simulink model "bh_smd_MAIN_simple"  (R2018a)
settings: configuration reference "CF_01" (kept outside this file)
settings Model: DataDictionary=MY_SMD_DATA_DICT.sldd  Creator=bhorton  LastModifiedBy=bhorton

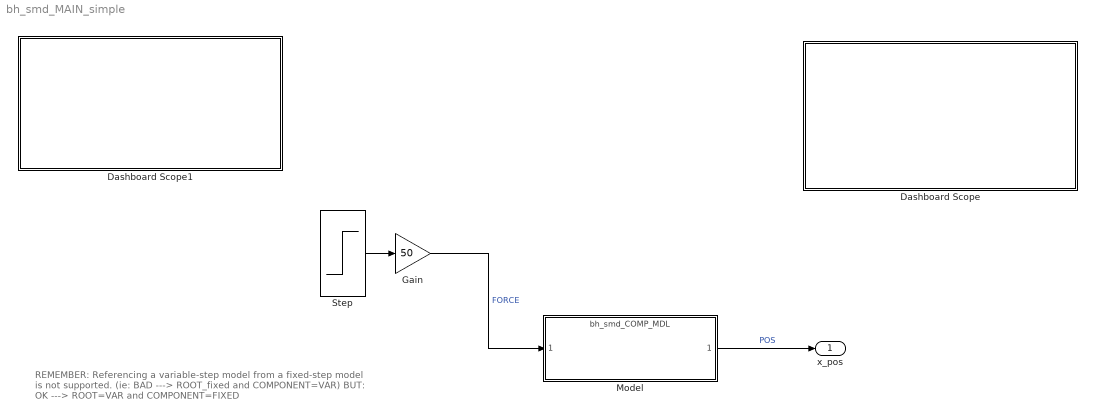
== system bh_smd_MAIN_simple ==
  note: REMEMBER:
      |
      | Referencing a variable-step model
      | from a fixed-step model is not supported.
      | (ie: BAD ---> ROOT_fixed and COMPONENT=VAR)
      |
      | BUT:
      | OK ---> ROOT=VAR and COMPONENT=FIXED
  Dashboard Scope : Subsystem  DialogController=hmiCreateDDGDialog  IsWebBlock=on  mask(MWDashboardBlock){webBlockId=47d7a76a-e090-4f37-bb13-c45fee118520, webBlockType=sdiscope, ShowInitialText=on, HMISrcModelName=bh_smd_MAIN_simple}
      mask prompts: webBlockId "WebBlock Id"; webBlockType "WebBlock Type"; HMISrcModelName "Source Model"
      mask help: SimulinkHMI:dialogs:HMIScopeDialogDesc
      mask Help: helpview([docroot '/mapfiles/simulink.map'], 'hmi_scope')
      mask Display:
      | if strcmp(get_param(bdroot(gcb),'BlockDiagramType'), 'library')
      |     image([(matlabroot) '/toolbox/simulink/hmi/icons/DashboardScope.png']);
      | end
  Dashboard Scope1 : Subsystem  DialogController=hmiCreateDDGDialog  IsWebBlock=on  mask(MWDashboardBlock){webBlockId=8ddedbd7-6b40-4d71-b8ad-862d34055e22, webBlockType=sdiscope, ShowInitialText=on, HMISrcModelName=bh_smd_MAIN_simple}
      mask prompts: webBlockId "WebBlock Id"; webBlockType "WebBlock Type"; HMISrcModelName "Source Model"
      mask help: SimulinkHMI:dialogs:HMIScopeDialogDesc
      mask Help: helpview([docroot '/mapfiles/simulink.map'], 'hmi_scope')
      mask Display:
      | if strcmp(get_param(bdroot(gcb),'BlockDiagramType'), 'library')
      |     image([(matlabroot) '/toolbox/simulink/hmi/icons/DashboardScope.png']);
      | end
  Gain : Gain  Gain=50
  Model : ModelReference  ModelNameDialog=bh_smd_COMP_MDL.slx  SimulationMode=Normal  ModelReferenceVersion=1.44
  Step : Step  Time=5  SampleTime=0
  x_pos : Outport
  wires:
  Step/1 -> Gain/1
  Gain/1 -> Model/1  "FORCE"
  Model/1 -> x_pos/1  "POS"

== system bh_smd_MAIN_simple/Dashboard Scope ==

== system bh_smd_MAIN_simple/Dashboard Scope1 ==
